simulink model "blinker_4_leds"  (R2015b)
settings: Solver=VariableStepAuto  StartTime=0.0  StopTime=inf  RelTol=1e-3
settings Model: Creator=scco1019  LastModifiedBy=scco1019

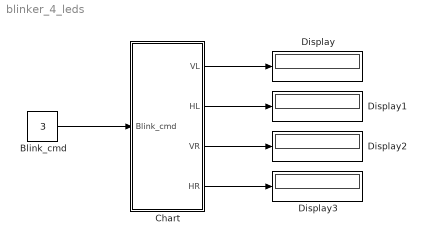
== system blinker_4_leds ==
  "Blink_cmd " : Constant  Value=3
  Chart : Stateflow chart  TreatAsAtomicUnit=on
  Display{,1..3} (4 alike) : Display
  wires:
  "Blink_cmd "/1 -> Chart/1(Blink_cmd)
  Chart/1(VL) -> Display/1
  Chart/2(HL) -> Display1/1
  Chart/3(VR) -> Display2/1
  Chart/4(HR) -> Display3/1

== stateflow chart blinker_4_leds/Chart ==
  state blinkidinki/
  (default) -> blinkidinki
  blinkidinki -> blinkidinki [order 4] : [Blink_cmd==0]
      | {HL=0;VL=0;HR=0;VR=0;}
  blinkidinki -> blinkidinki [order 1] : [Blink_cmd==2]
      | {HL=0;VL=0;HR=1;VR=1;}
  blinkidinki -> blinkidinki [order 3] : [Blink_cmd==1]
      | {HL=1;VL=1;HR=0;VR=0;}
  blinkidinki -> blinkidinki [order 2] : [Blink_cmd==3]
      | {HL=1;VL=1;HR=1;VR=1;}
  data: Blink_cmd input; VL output; HL output; VR output; HR output
